simulink model "sim_robot_nocontrol"  (R2019b)
settings: Solver=VariableStepAuto  StartTime=0.0  StopTime=T_tot  FixedStep=0.0001  RelTol=1e-3
model workspace: external: MATLAB File G:\Drive condivisi\SSR_project\cad\modello_ultimo\sim\robot_DataFile.m (data not in the file)
undefined symbols (not defined in the file or in its folder): sigbuilder_block, smiData, X, Y, Z
libraries: sm_lib x40, nesl_utility x28
(part 2 of 2)

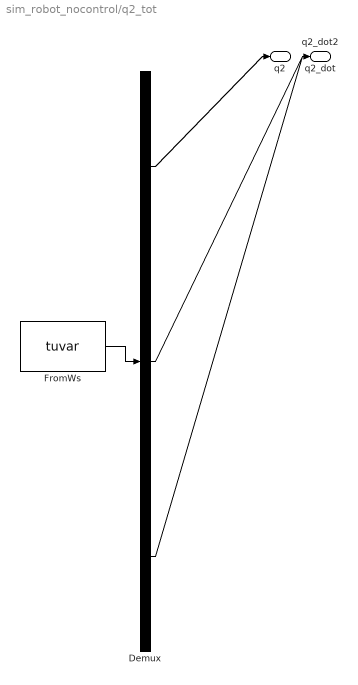
== system sim_robot_nocontrol/q2_tot ==
  Demux : Demux  Tag=STV Demux  Outputs=3
  FromWs : FromWorkspace  Tag=STV FromWs  VariableName=tuvar  SampleTime=0
      SigBuilderData=|
      | common.afterFinalStr = 'Extrapolate'
      | common.sampleTime = 0
      | dataSet.timeRange = [0 57.824]
      | dataSet.name = 'Group 1'
      | sbobj.Groups.Name = 'Group 1'
      | sbobj.Groups.Signals(1).Name = 'q2'
      | sbobj.Groups.Signals(1).XData = [0 0.0505050505051 0.10101010101 0.151515151515 0.20202020202 0.252525252525 0.30303030303 0.353535353535 0.40404040404 0.454545454545 0.505050505051 0.555555555556 ... (1981 elements, 1x1981)]
      | sbobj.Groups.Signals(1).YData = [0 0 0 0 0 0 0 0 0 0 0 0 ... (1981 elements, 1x1981)]
      | sbobj.Groups.Signals(2).Name = 'q2_dot'
      | sbobj.Groups.Signals(2).XData = [0 0.0505050505051 0.10101010101 0.151515151515 0.20202020202 0.252525252525 0.30303030303 0.353535353535 0.40404040404 0.454545454545 0.505050505051 0.555555555556 ... (1981 elements, 1x1981)]
      | sbobj.Groups.Signals(2).YData = [0 0 0 0 0 0 0 0 0 0 0 0 ... (1981 elements, 1x1981)]
      | sbobj.Groups.Signals(3).Name = 'q2_dot2'
      | sbobj.Groups.Signals(3).XData = [0 0.0505050505051 0.10101010101 0.151515151515 0.20202020202 0.252525252525 0.30303030303 0.353535353535 0.40404040404 0.454545454545 0.505050505051 0.555555555556 ... (1981 elements, 1x1981)]
      | sbobj.Groups.Signals(3).YData = [0 0 0 0 0 0 0 0 0 0 0 0 ... (1981 elements, 1x1981)]
      | sbobj.Groups.TimeRange = [0 57.824]
  q2 : Outport  Tag=STV Outport
  q2_dot : Outport  Tag=STV Outport  Port=2
  q2_dot2 : Outport  Tag=STV Outport  Port=3
  wires:
  FromWs/1 -> Demux/1
  Demux/1 -> q2/1
  Demux/2 -> q2_dot/1
  Demux/3 -> q2_dot2/1

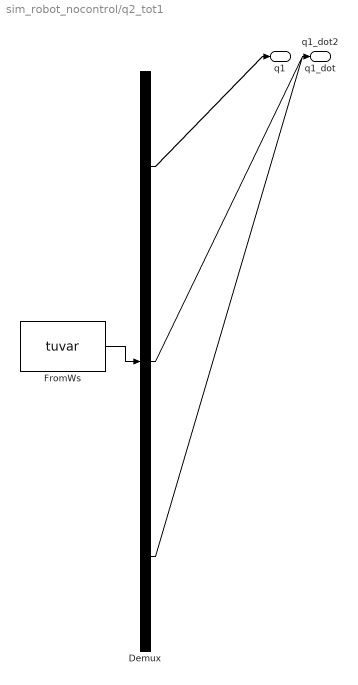
== system sim_robot_nocontrol/q2_tot1 ==
  Demux : Demux  Tag=STV Demux  Outputs=3
  FromWs : FromWorkspace  Tag=STV FromWs  VariableName=tuvar  SampleTime=0
      SigBuilderData=|
      | common.afterFinalStr = 'Extrapolate'
      | common.sampleTime = 0
      | dataSet.timeRange = [0 57.824]
      | dataSet.name = 'Group 1'
      | sbobj.Groups.Name = 'Group 1'
      | sbobj.Groups.Signals(1).Name = 'q1'
      | sbobj.Groups.Signals(1).XData = [0 0.0505050505051 0.10101010101 0.151515151515 0.20202020202 0.252525252525 0.30303030303 0.353535353535 0.40404040404 0.454545454545 0.505050505051 0.555555555556 ... (1981 elements, 1x1981)]
      | sbobj.Groups.Signals(1).YData = [0 0 0 0 0 0 0 0 0 0 0 0 ... (1981 elements, 1x1981)]
      | sbobj.Groups.Signals(2).Name = 'q1_dot'
      | sbobj.Groups.Signals(2).XData = [0 0.0505050505051 0.10101010101 0.151515151515 0.20202020202 0.252525252525 0.30303030303 0.353535353535 0.40404040404 0.454545454545 0.505050505051 0.555555555556 ... (1981 elements, 1x1981)]
      | sbobj.Groups.Signals(2).YData = [0 0 0 0 0 0 0 0 0 0 0 0 ... (1981 elements, 1x1981)]
      | sbobj.Groups.Signals(3).Name = 'q1_dot2'
      | sbobj.Groups.Signals(3).XData = [0 0.0505050505051 0.10101010101 0.151515151515 0.20202020202 0.252525252525 0.30303030303 0.353535353535 0.40404040404 0.454545454545 0.505050505051 0.555555555556 ... (1981 elements, 1x1981)]
      | sbobj.Groups.Signals(3).YData = [0 0 0 0 0 0 0 0 0 0 0 0 ... (1981 elements, 1x1981)]
      | sbobj.Groups.TimeRange = [0 57.824]
  q1 : Outport  Tag=STV Outport
  q1_dot : Outport  Tag=STV Outport  Port=2
  q1_dot2 : Outport  Tag=STV Outport  Port=3
  wires:
  FromWs/1 -> Demux/1
  Demux/1 -> q1/1
  Demux/2 -> q1_dot/1
  Demux/3 -> q1_dot2/1

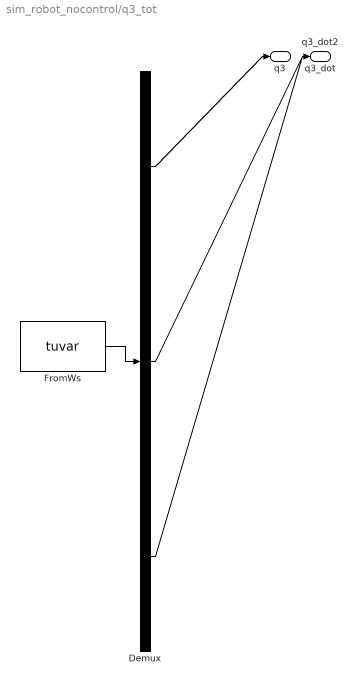
== system sim_robot_nocontrol/q3_tot ==
  Demux : Demux  Tag=STV Demux  Outputs=3
  FromWs : FromWorkspace  Tag=STV FromWs  VariableName=tuvar  SampleTime=0
      SigBuilderData=|
      | common.afterFinalStr = 'Extrapolate'
      | common.sampleTime = 0
      | dataSet.timeRange = [0 57.824]
      | dataSet.name = 'Group 1'
      | sbobj.Groups.Name = 'Group 1'
      | sbobj.Groups.Signals(1).Name = 'q3'
      | sbobj.Groups.Signals(1).XData = [0 0.0505050505051 0.10101010101 0.151515151515 0.20202020202 0.252525252525 0.30303030303 0.353535353535 0.40404040404 0.454545454545 0.505050505051 0.555555555556 ... (1981 elements, 1x1981)]
      | sbobj.Groups.Signals(1).YData = [0 0 0 0 0 0 0 0 0 0 0 0 ... (1981 elements, 1x1981)]
      | sbobj.Groups.Signals(2).Name = 'q3_dot'
      | sbobj.Groups.Signals(2).XData = [0 0.0505050505051 0.10101010101 0.151515151515 0.20202020202 0.252525252525 0.30303030303 0.353535353535 0.40404040404 0.454545454545 0.505050505051 0.555555555556 ... (1981 elements, 1x1981)]
      | sbobj.Groups.Signals(2).YData = [0 0 0 0 0 0 0 0 0 0 0 0 ... (1981 elements, 1x1981)]
      | sbobj.Groups.Signals(3).Name = 'q3_dot2'
      | sbobj.Groups.Signals(3).XData = [0 0.0505050505051 0.10101010101 0.151515151515 0.20202020202 0.252525252525 0.30303030303 0.353535353535 0.40404040404 0.454545454545 0.505050505051 0.555555555556 ... (1981 elements, 1x1981)]
      | sbobj.Groups.Signals(3).YData = [0 0 0 0 0 0 0 0 0 0 0 0 ... (1981 elements, 1x1981)]
      | sbobj.Groups.TimeRange = [0 57.824]
  q3 : Outport  Tag=STV Outport
  q3_dot : Outport  Tag=STV Outport  Port=2
  q3_dot2 : Outport  Tag=STV Outport  Port=3
  wires:
  FromWs/1 -> Demux/1
  Demux/1 -> q3/1
  Demux/2 -> q3_dot/1
  Demux/3 -> q3_dot2/1
